simulink model "RFB_parasitic_method"  (R2020a)
settings: Solver=VariableStepAuto  StartTime=0.0  StopTime=10.0  RelTol=1e-3
undefined symbols (not defined in the file or in its folder): relay_params, ts
settings Model: Creator=rshousha  LastModifiedBy=jwai
settings DataIOCC: ReturnWorkspaceOutputs=off
settings DebuggingCC: ArithmeticOperatorsInVariantConditions=warning
settings SFSimCC: CustomCodeUndefinedFunction=UseInterfaceOnly

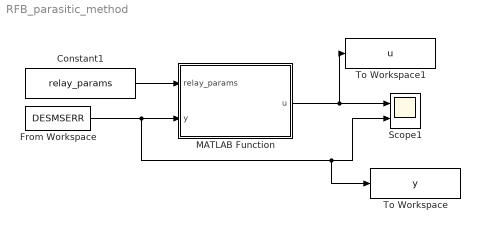
== system RFB_parasitic_method ==
  Constant1 : Constant  Value=relay_params
  From Workspace : FromWorkspace  VariableName=DESMSERR  SampleTime=[ts]
  MATLAB Function : MATLAB Function  TreatAsAtomicUnit=on
  Scope1 : Scope  NumInputPorts=2
  To Workspace : ToWorkspace  VariableName=y  SaveFormat=Timeseries  SampleTime=-1
  To Workspace1 : ToWorkspace  VariableName=u  SaveFormat=Timeseries  SampleTime=-1
      settings: Save2DSignal=2-D array (concatenate along first dimension)
  wires:
  Constant1/1 -> MATLAB Function/1(relay_params)
  From Workspace/1 -> To Workspace/1, Scope1/2, MATLAB Function/2(y)
  MATLAB Function/1(u) -> To Workspace1/1, Scope1/1

== matlab function RFB_parasitic_method/MATLAB Function ==
  data: relay_params input; y input; u output
function u  = parasitic_relay(relay_params, y)

persistent urelays_km1

d = relay_params(1);
output_bias_frac = relay_params(2);
input_bias = relay_params(3);
hysteresis = relay_params(4);
nparasites = relay_params(5);
alpha = relay_params(6:(5+nparasites));

beta = [1; alpha];  % multipliers for relays, including base relay

urelays = zeros(size(beta));
if isempty(urelays_km1)
  urelays = beta * d;
  urelays_km1 = urelays;
end

%% Base relay
if     (y > -input_bias + hysteresis)
    urelays(1) = d;
elseif (y < -input_bias - hysteresis)
    urelays(1) = -d;
else
    urelays(1) = urelays_km1(1);
end

%% Parasitic relays
for i = 2:length(beta)
  if (urelays_km1(i-1) > 0) && (urelays(i-1) < 0)
    urelays(i) = -beta(i) * d * sign(urelays_km1(i));
  else
    urelays(i) = urelays_km1(i);
  end
end

urelays_km1 = urelays;

%% Combined output with output bias
u = sum(urelays) + output_bias_frac * d;
    
    
end
